simulink model "undirect_graph_disturbance_TBG"  (R2020a)
settings: Solver=FixedStepAuto  StartTime=0.0  StopTime=10.0  FixedStep=0.0001  RelTol=1e-3
libraries: simulink x10
settings Model: Creator=WangQipeng  LastModifiedBy=WangQipeng

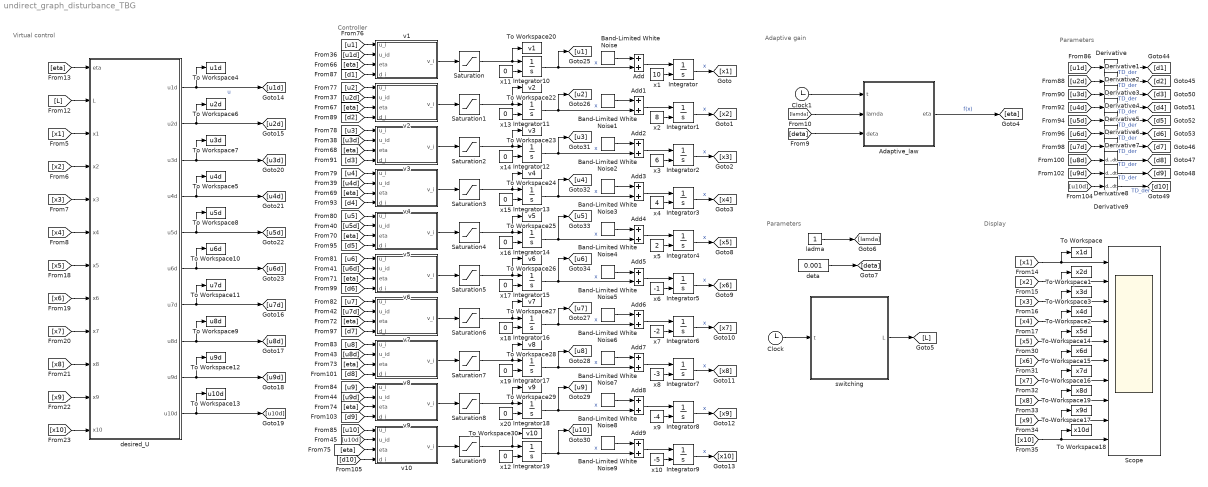
== system undirect_graph_disturbance_TBG ==
  note: Virtual control
  note: Controller
  note: Display
  note: Parameters
  note: Adaptive gain
  note: Parameters
  Adaptive_law : MATLAB Function  TreatAsAtomicUnit=on
  Add{,1..9} (10 alike) : Sum
  Band-Limited White Noise : simulink/Sources/Band-Limited White Noise  Cov=[0.01]  Ts=0.01  seed=[23341]
  Band-Limited White Noise1 : simulink/Sources/Band-Limited White Noise  Cov=[0.01]  Ts=0.01  seed=[22141]
  Band-Limited White Noise2 : simulink/Sources/Band-Limited White Noise  Cov=[0.01]  Ts=0.01  seed=[27541]
  Band-Limited White Noise3 : simulink/Sources/Band-Limited White Noise  Cov=[0.01]  Ts=0.01  seed=[23841]
  Band-Limited White Noise4 : simulink/Sources/Band-Limited White Noise  Cov=[0.01]  Ts=0.01  seed=[25341]
  Band-Limited White Noise5 : simulink/Sources/Band-Limited White Noise  Cov=[0.01]  Ts=0.01  seed=[23261]
  Band-Limited White Noise6 : simulink/Sources/Band-Limited White Noise  Cov=[0.01]  Ts=0.01  seed=[21241]
  Band-Limited White Noise7 : simulink/Sources/Band-Limited White Noise  Cov=[0.01]  Ts=0.01  seed=[27841]
  Band-Limited White Noise8 : simulink/Sources/Band-Limited White Noise  Cov=[0.01]  Ts=0.01  seed=[23361]
  Band-Limited White Noise9 : simulink/Sources/Band-Limited White Noise  Cov=[0.01]  Ts=0.01  seed=[23521]
  Clock : Clock
  Clock1 : Clock
  Derivative{,1..9} (10 alike) : Derivative
  Integrator{,1..19} (20 alike) : Integrator  InitialConditionSource=external  InitialCondition=1
  Saturation{,1..9} (10 alike) : Saturate  UpperLimit=30  LowerLimit=-30
  Scope : Scope  NumInputPorts=10
  To Workspace : ToWorkspace  VariableName=x1d  SaveFormat=Timeseries  SampleTime=-1
  To Workspace1 : ToWorkspace  VariableName=x2d  SaveFormat=Timeseries  SampleTime=-1
  To Workspace10 : ToWorkspace  VariableName=u6d  SaveFormat=Timeseries  SampleTime=-1
  To Workspace11 : ToWorkspace  VariableName=u7d  SaveFormat=Timeseries  SampleTime=-1
  To Workspace12 : ToWorkspace  VariableName=u9d  SaveFormat=Timeseries  SampleTime=-1
  To Workspace13 : ToWorkspace  VariableName=u10d  SaveFormat=Timeseries  SampleTime=-1
  To Workspace14 : ToWorkspace  VariableName=x5d  SaveFormat=Timeseries  SampleTime=-1
  To Workspace15 : ToWorkspace  VariableName=x6d  SaveFormat=Timeseries  SampleTime=-1
  To Workspace16 : ToWorkspace  VariableName=x7d  SaveFormat=Timeseries  SampleTime=-1
  To Workspace17 : ToWorkspace  VariableName=x9d  SaveFormat=Timeseries  SampleTime=-1
  To Workspace18 : ToWorkspace  VariableName=x10d  SaveFormat=Timeseries  SampleTime=-1
  To Workspace19 : ToWorkspace  VariableName=x8d  SaveFormat=Timeseries  SampleTime=-1
  To Workspace2 : ToWorkspace  VariableName=x4d  SaveFormat=Timeseries  SampleTime=-1
  To Workspace20 : ToWorkspace  VariableName=v1  SaveFormat=Timeseries  SampleTime=-1
  To Workspace22 : ToWorkspace  VariableName=v2  SaveFormat=Timeseries  SampleTime=-1
  To Workspace23 : ToWorkspace  VariableName=v3  SaveFormat=Timeseries  SampleTime=-1
  To Workspace24 : ToWorkspace  VariableName=v4  SaveFormat=Timeseries  SampleTime=-1
  To Workspace25 : ToWorkspace  VariableName=v5  SaveFormat=Timeseries  SampleTime=-1
  To Workspace26 : ToWorkspace  VariableName=v6  SaveFormat=Timeseries  SampleTime=-1
  To Workspace27 : ToWorkspace  VariableName=v7  SaveFormat=Timeseries  SampleTime=-1
  To Workspace28 : ToWorkspace  VariableName=v8  SaveFormat=Timeseries  SampleTime=-1
  To Workspace29 : ToWorkspace  VariableName=v9  SaveFormat=Timeseries  SampleTime=-1
  To Workspace3 : ToWorkspace  VariableName=x3d  SaveFormat=Timeseries  SampleTime=-1
  To Workspace30 : ToWorkspace  VariableName=v10  SaveFormat=Timeseries  SampleTime=-1
  To Workspace4 : ToWorkspace  VariableName=u1d  SaveFormat=Timeseries  SampleTime=-1
  To Workspace5 : ToWorkspace  VariableName=u4d  SaveFormat=Timeseries  SampleTime=-1
  To Workspace6 : ToWorkspace  VariableName=u2d  SaveFormat=Timeseries  SampleTime=-1
  To Workspace7 : ToWorkspace  VariableName=u3d  SaveFormat=Timeseries  SampleTime=-1
  To Workspace8 : ToWorkspace  VariableName=u5d  SaveFormat=Timeseries  SampleTime=-1
  To Workspace9 : ToWorkspace  VariableName=u8d  SaveFormat=Timeseries  SampleTime=-1
  desired_U : MATLAB Function  TreatAsAtomicUnit=on
  deta : Constant  Value=0.001
  ladma : Constant
  switching : MATLAB Function  TreatAsAtomicUnit=on
  v1 : MATLAB Function  TreatAsAtomicUnit=on
  v10 : MATLAB Function  TreatAsAtomicUnit=on
  v2 : MATLAB Function  TreatAsAtomicUnit=on
  v3 : MATLAB Function  TreatAsAtomicUnit=on
  v4 : MATLAB Function  TreatAsAtomicUnit=on
  v5 : MATLAB Function  TreatAsAtomicUnit=on
  v6 : MATLAB Function  TreatAsAtomicUnit=on
  v7 : MATLAB Function  TreatAsAtomicUnit=on
  v8 : MATLAB Function  TreatAsAtomicUnit=on
  v9 : MATLAB Function  TreatAsAtomicUnit=on
  x1 : Constant  Value=10
  x10 : Constant  Value=-5
  x{11..20} (10 alike) : Constant  Value=0
  x2 : Constant  Value=8
  x3 : Constant  Value=6
  x4 : Constant  Value=4
  x5 : Constant  Value=2
  x6 : Constant  Value=-1
  x7 : Constant  Value=-2
  x8 : Constant  Value=-3
  x9 : Constant  Value=-4
  wires:
  Integrator/1 -> [x1]  "x"
  Integrator1/1 -> [x2]  "x"
  Integrator2/1 -> [x3]  "x"
  Integrator3/1 -> [x4]  "x"
  [x3] -> desired_U/5(x3)
  [x4] -> desired_U/6(x4)
  [x1] -> desired_U/3(x1)
  [x2] -> desired_U/4(x2)
  [L] -> desired_U/2(L)
  [eta] -> desired_U/1(eta)
  x1/1 -> Integrator/2
  x2/1 -> Integrator1/2
  x3/1 -> Integrator2/2
  x4/1 -> Integrator3/2
  [x1] -> To Workspace/1, Scope/1
  [x2] -> To Workspace1/1, Scope/2
  [x3] -> To Workspace3/1, Scope/3
  [x4] -> To Workspace2/1, Scope/4
  Band-Limited White Noise/1 -> Add/1
  Add/1 -> Integrator/1
  Band-Limited White Noise1/1 -> Add1/1
  Add1/1 -> Integrator1/1
  Band-Limited White Noise2/1 -> Add2/1
  Add2/1 -> Integrator2/1
  Add3/1 -> Integrator3/1
  Band-Limited White Noise3/1 -> Add3/1
  Add7/1 -> Integrator7/1
  x7/1 -> Integrator6/2
  Band-Limited White Noise5/1 -> Add5/1
  Integrator7/1 -> [x8]  "x"
  x6/1 -> Integrator5/2
  x8/1 -> Integrator7/2
  Add6/1 -> Integrator6/1
  Add5/1 -> Integrator5/1
  Add4/1 -> Integrator4/1
  x5/1 -> Integrator4/2
  Band-Limited White Noise7/1 -> Add7/1
  Integrator4/1 -> [x5]  "x"
  Integrator6/1 -> [x7]  "x"
  Band-Limited White Noise6/1 -> Add6/1
  Integrator5/1 -> [x6]  "x"
  Band-Limited White Noise4/1 -> Add4/1
  Band-Limited White Noise9/1 -> Add9/1
  x10/1 -> Integrator9/2
  Add9/1 -> Integrator9/1
  Add8/1 -> Integrator8/1
  x9/1 -> Integrator8/2
  Integrator8/1 -> [x9]  "x"
  Integrator9/1 -> [x10]  "x"
  Band-Limited White Noise8/1 -> Add8/1
  [x10] -> desired_U/12(x10)
  [x9] -> desired_U/11(x9)
  [x8] -> desired_U/10(x8)
  [x7] -> desired_U/9(x7)
  [x6] -> desired_U/8(x6)
  [x5] -> desired_U/7(x5)
  [x6] -> To Workspace15/1, Scope/6
  [x7] -> To Workspace16/1, Scope/7
  [x8] -> To Workspace19/1, Scope/8
  [x5] -> To Workspace14/1, Scope/5
  [x10] -> To Workspace18/1, Scope/10
  [x9] -> To Workspace17/1, Scope/9
  switching/1(L) -> [L]
  Clock/1 -> switching/1(t)
  x15/1 -> Integrator13/2
  v8/1(v_i) -> Saturation7/1
  v7/1(v_i) -> Saturation6/1
  x19/1 -> Integrator17/2
  x17/1 -> Integrator15/2
  v1/1(v_i) -> Saturation/1
  v6/1(v_i) -> Saturation5/1
  v2/1(v_i) -> Saturation1/1
  v3/1(v_i) -> Saturation2/1
  x18/1 -> Integrator16/2
  x16/1 -> Integrator14/2
  x13/1 -> Integrator11/2
  x14/1 -> Integrator12/2
  x12/1 -> Integrator19/2
  v4/1(v_i) -> Saturation3/1
  v10/1(v_i) -> Saturation9/1
  v5/1(v_i) -> Saturation4/1
  v9/1(v_i) -> Saturation8/1
  x20/1 -> Integrator18/2
  x11/1 -> Integrator10/2
  Integrator10/1 -> [u1], Add/2  "x"
  Integrator11/1 -> [u2], Add1/2  "x"
  Integrator12/1 -> [u3], Add2/2  "x"
  Integrator13/1 -> [u4], Add3/2  "x"
  Integrator14/1 -> [u5], Add4/2  "x"
  Integrator15/1 -> [u6], Add5/2  "x"
  Integrator16/1 -> [u7], Add6/2  "x"
  Integrator17/1 -> [u8], Add7/2  "x"
  Integrator18/1 -> [u9], Add8/2  "x"
  Integrator19/1 -> [u10], Add9/2  "x"
  desired_U/1(u1d) -> To Workspace4/1, [u1d]  "u"
  desired_U/2(u2d) -> To Workspace6/1, [u2d]
  desired_U/3(u3d) -> To Workspace7/1, [u3d]
  desired_U/4(u4d) -> To Workspace5/1, [u4d]
  desired_U/5(u5d) -> To Workspace8/1, [u5d]
  desired_U/6(u6d) -> To Workspace10/1, [u6d]
  desired_U/7(u7d) -> To Workspace11/1, [u7d]
  desired_U/8(u8d) -> To Workspace9/1, [u8d]
  desired_U/9(u9d) -> To Workspace12/1, [u9d]
  desired_U/10(u10d) -> To Workspace13/1, [u10d]
  [u1d] -> v1/2(u_id)
  [u1] -> v1/1(u_i)
  [eta] -> v1/3(eta)
  [u2] -> v2/1(u_i)
  [u2d] -> v2/2(u_id)
  [eta] -> v2/3(eta)
  [eta] -> v6/3(eta)
  [eta] -> v7/3(eta)
  [eta] -> v8/3(eta)
  [eta] -> v9/3(eta)
  [u10] -> v10/1(u_i)
  [u8d] -> v8/2(u_id)
  [u8] -> v8/1(u_i)
  [u7d] -> v7/2(u_id)
  [u7] -> v7/1(u_i)
  [u6d] -> v6/2(u_id)
  [u6] -> v6/1(u_i)
  [eta] -> v5/3(eta)
  [u5d] -> v5/2(u_id)
  [u5] -> v5/1(u_i)
  [eta] -> v4/3(eta)
  [u4d] -> v4/2(u_id)
  [u4] -> v4/1(u_i)
  [eta] -> v3/3(eta)
  [u3d] -> v3/2(u_id)
  [u3] -> v3/1(u_i)
  [u9] -> v9/1(u_i)
  [u9d] -> v9/2(u_id)
  [u10d] -> v10/2(u_id)
  [eta] -> v10/3(eta)
  [u10d] -> Derivative9/1
  [u9d] -> Derivative8/1
  [u8d] -> Derivative7/1
  [u7d] -> Derivative6/1
  [u6d] -> Derivative5/1
  [u5d] -> Derivative4/1
  [u4d] -> Derivative3/1
  [u3d] -> Derivative2/1
  [u2d] -> Derivative1/1
  [u1d] -> Derivative/1
  Derivative/1 -> [d1]  "TD_der"
  Derivative1/1 -> [d2]  "TD_der"
  Derivative2/1 -> [d3]  "TD_der"
  Derivative3/1 -> [d4]  "TD_der"
  Derivative4/1 -> [d5]  "TD_der"
  Derivative5/1 -> [d6]  "TD_der"
  Derivative6/1 -> [d7]  "TD_der"
  Derivative7/1 -> [d8]  "TD_der"
  Derivative8/1 -> [d9]  "TD_der"
  Derivative9/1 -> [d10]  "TD_der"
  [d10] -> v10/4(d_i)
  [d9] -> v9/4(d_i)
  [d8] -> v8/4(d_i)
  [d7] -> v7/4(d_i)
  [d6] -> v6/4(d_i)
  [d5] -> v5/4(d_i)
  [d4] -> v4/4(d_i)
  [d3] -> v3/4(d_i)
  [d2] -> v2/4(d_i)
  [d1] -> v1/4(d_i)
  [lamda] -> Adaptive_law/2(lamda)
  Clock1/1 -> Adaptive_law/1(t)
  Adaptive_law/1(eta) -> [eta]  "f(x)"
  [deta] -> Adaptive_law/3(deta)
  deta/1 -> [deta]
  ladma/1 -> [lamda]
  Saturation/1 -> To Workspace20/1, Integrator10/1
  Saturation1/1 -> To Workspace22/1, Integrator11/1
  Saturation2/1 -> To Workspace23/1, Integrator12/1
  Saturation3/1 -> To Workspace24/1, Integrator13/1
  Saturation4/1 -> To Workspace25/1, Integrator14/1
  Saturation5/1 -> To Workspace26/1, Integrator15/1
  Saturation6/1 -> To Workspace27/1, Integrator16/1
  Saturation7/1 -> To Workspace28/1, Integrator17/1
  Saturation8/1 -> To Workspace29/1, Integrator18/1
  Saturation9/1 -> To Workspace30/1, Integrator19/1

== matlab function undirect_graph_disturbance_TBG/v4 ==
  data: u_i input; v_i output; u_id input; eta input; d_i input
function v_i  = protocol(u_i,u_id,eta,d_i)
v_i = d_i -(eta + 1) * (u_i - u_id);

== matlab function undirect_graph_disturbance_TBG/v5 ==
  data: u_i input; v_i output; u_id input; eta input; d_i input
function v_i  = protocol(u_i,u_id,eta,d_i)
v_i = d_i -(eta + 1) * (u_i - u_id);

== matlab function undirect_graph_disturbance_TBG/v10 ==
  data: u_i input; v_i output; u_id input; eta input; d_i input
function v_i  = protocol(u_i,u_id,eta,d_i)
v_i = d_i -(eta + 1) * (u_i - u_id);

== matlab function undirect_graph_disturbance_TBG/v6 ==
  data: u_i input; v_i output; u_id input; eta input; d_i input
function v_i  = protocol(u_i,u_id,eta,d_i)
v_i = d_i -(eta + 1) * (u_i - u_id);

== matlab function undirect_graph_disturbance_TBG/v7 ==
  data: u_i input; v_i output; u_id input; eta input; d_i input
function v_i  = protocol(u_i,u_id,eta,d_i)
v_i = d_i -(eta + 1) * (u_i - u_id);

== matlab function undirect_graph_disturbance_TBG/v8 ==
  data: u_i input; v_i output; u_id input; eta input; d_i input
function v_i  = protocol(u_i,u_id,eta,d_i)
v_i = d_i -(eta + 1) * (u_i - u_id);

== matlab function undirect_graph_disturbance_TBG/v9 ==
  data: u_i input; v_i output; u_id input; eta input; d_i input
function v_i  = protocol(u_i,u_id,eta,d_i)
v_i = d_i -(eta + 1) * (u_i - u_id);

== matlab function undirect_graph_disturbance_TBG/desired_U ==
  data: eta input; u1d output; L input; x1 input; x2 input; x3 input; x4 input; u2d output; u3d output; u4d output; x5 input; x6 input; x7 input; x8 input; x9 input; x10 input; u5d output; u6d output; u7d output; u8d output; u9d output; u10d output
function [u1d,u2d,u3d,u4d,u5d,u6d,u7d,u8d,u9d,u10d] = First_order_protocol(eta,L,x1,x2,x3,x4,x5,x6,x7,x8,x9,x10)
x = [x1;x2;x3;x4;x5;x6;x7;x8;x9;x10];
temp = -(eta + 1) * L * x;


u1d = temp(1);
u2d = temp(2);
u3d = temp(3);
u4d = temp(4);
u5d = temp(5);
u6d = temp(6);
u7d = temp(7);
u8d = temp(8);
u9d = temp(9);
u10d = temp(10);

== matlab function undirect_graph_disturbance_TBG/Adaptive_law ==
  data: t input; eta output; lamda input; deta input
function eta = TBG(t,lamda,deta)
if(t<=4)
    zeta = 10/(4^6)*t^6 - 24/(4^5)*t^5 + 15/(4^4)*t^4;
    d_zeta = 60/(4^6)*t^5 - 120/(4^5)*t^4 + 15/(4^3)*t^3;
else
    zeta = 1;
    d_zeta = 0;
end

eta = d_zeta/(2 * lamda * (1 - zeta + deta));

== matlab function undirect_graph_disturbance_TBG/switching ==
  data: t input; L output
function L = Switch(t)
if t<1
    L = 0.5*[2 -1 0 0 0 0 0 0 0 -1;
 -1 2 -1 0 0 0 0 0 0 0;
 0 -1 2 -1 0 0 0 0 0 0;
 0 0 -1 2 -1 0 0 0 0 0;
 0 0 0 -1 2 -1 0 0 0 0;
 0 0 0 0 -1 2 -1 0 0 0;
 0 0 0 0 0 -1 2 -1 0 0;
 0 0 0 0 0 0 -1 2 -1 0;
 0 0 0 0 0 0 0 -1 2 -1;
 -1 0 0 0 0 0 0 0 -1 2];
elseif t<6
    L = [3 0 0 -1 0 -1 0 -1 0 0;
 0 3 0 0 -1 0 -1 0 -1 0;
 0 0 3 0 0 -1 0 -1 0 -1;
 -1 0 0 3 0 0 -1 0 -1 0;
 0 -1 0 0 3 0 0 -1 0 -1;
 -1 0 -1 0 0 3 0 0 -1 0;
 0 -1 0 -1 0 0 3 0 0 -1;
 -1 0 -1 0 -1 0 0 3 0 0;
 0 -1 0 -1 0 -1 0 0 3 0;
 0 0 -1 0 -1 0 -1 0 0 3];
else
    L = 0.5*[2 -1 0 0 0 0 0 0 0 -1;
 -1 2 -1 0 0 0 0 0 0 0;
 0 -1 2 -1 0 0 0 0 0 0;
 0 0 -1 2 -1 0 0 0 0 0;
 0 0 0 -1 2 -1 0 0 0 0;
 0 0 0 0 -1 2 -1 0 0 0;
 0 0 0 0 0 -1 2 -1 0 0;
 0 0 0 0 0 0 -1 2 -1 0;
 0 0 0 0 0 0 0 -1 2 -1;
 -1 0 0 0 0 0 0 0 -1 2];
end

== matlab function undirect_graph_disturbance_TBG/v1 ==
  data: u_i input; v_i output; u_id input; eta input; d_i input
function v_i  = protocol(u_i,u_id,eta,d_i)
v_i = d_i -(eta + 1) * (u_i - u_id);

== matlab function undirect_graph_disturbance_TBG/v2 ==
  data: u_i input; v_i output; u_id input; eta input; d_i input
function v_i  = protocol(u_i,u_id,eta,d_i)
v_i = d_i -(eta + 1) * (u_i - u_id);

== matlab function undirect_graph_disturbance_TBG/v3 ==
  data: u_i input; v_i output; u_id input; eta input; d_i input
function v_i  = protocol(u_i,u_id,eta,d_i)
v_i = d_i -(eta + 1) * (u_i - u_id);
